simulink model "fengji"  (R2022b)
settings: Solver=VariableStepAuto  StartTime=0.0  StopTime=1.2  RelTol=1e-3
InitFcn:
  | Udc=311;
  | R=0.958;
  | Ld=5.25e-3;
  | Lq=12e-3;
  | flux=0.1827;
  | J=0.003;
  | B=0.008;
  | Pn=4;
  | Kpd=1100*0.958;
  | Kid=1100*R;
  | Kpq=1100*Lq;
  | Kiq=1100*R;
  | uppermin=-311*0.9*sqrt(1/3);
  | uppermax=311*0.9*sqrt(1/3);
  | uppermin2=-311*0.9*sqrt(1/3);
  | uppermax2=311*0.9*sqrt(1/3);
  | Kpw=0.14;
  | Kiw=0.14*50;
  | Ba=0.013;
undefined symbols (not defined in the file): DiscIntNeverNeededParam
libraries: simulink x11, slpidlib x6, spsabctodq0Lib x3, spsUniversalBridgeLib x3, spsPermanentMagnetSynchronousMachineLib x2, spsSVPWMGenerator2LevelLib x2, spsdq0toAlphaBetaZeroLib x2, spsPower3phInstantaneousLib x1, spsPower3phPhasorLib x1, spsSeriesRLCBranchLib x1, spsDCVoltageSourceLib x1, spsThreePhaseSeriesRLCBranchLib x1
(part 1 of 2)
settings Model: SimulationMode=accelerator  Creator=V V  LastModifiedBy=58239
settings SolverCC: AlgebraicLoopSolver=TrustRegion
settings OptimizationCC: LifeSpan=inf
settings DebuggingCC: UnconnectedInputMsg=warning  UnconnectedOutputMsg=warning  UnconnectedLineMsg=warning  SFExecutionAtInitializationDiag=none  SFMachineParentedDataDiag=warning  ArithmeticOperatorsInVariantConditions=warning
settings ModelReferenceCC: EnableRefExpFcnMdlSchedulingChecks=on
settings SFSimCC: CustomCodeUndefinedFunction=UseInterfaceOnly
settings CodeAppCC: StateflowObjectComments=on

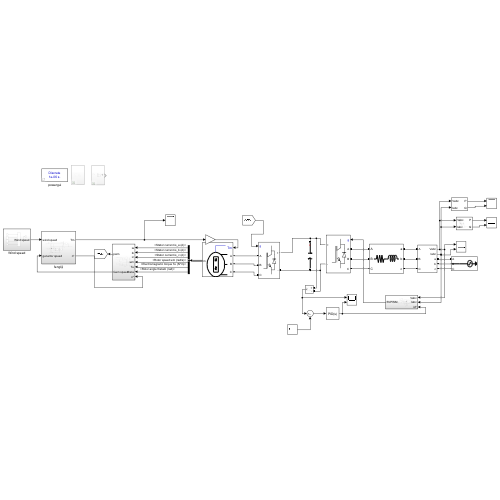
[thumbnail: Simulink's stored preview of the top-level diagram]
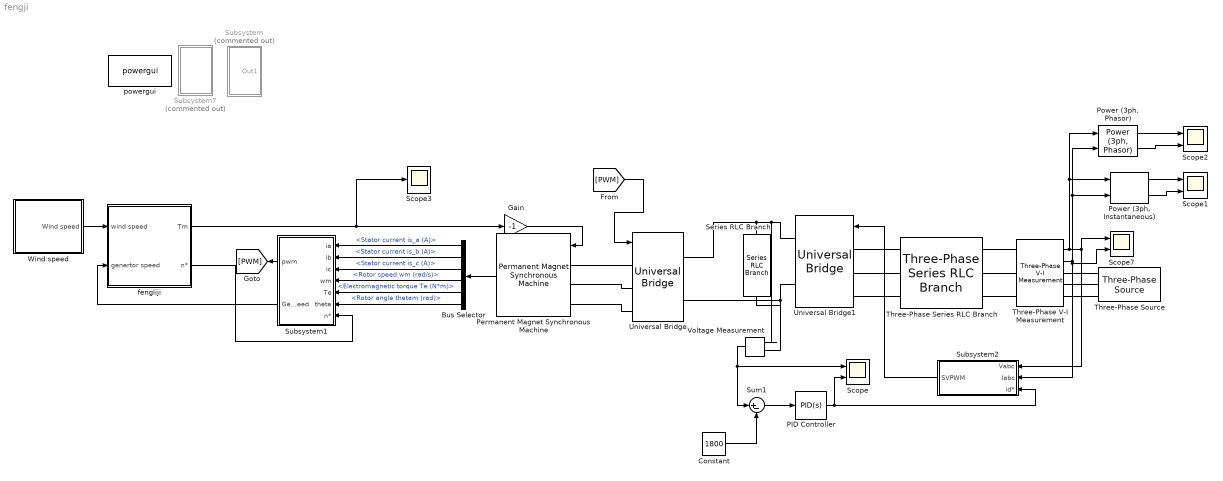
== system fengji ==
  Bus Selector : BusSelector  OutputSignals=Stator current is_a (A),Stator current is_b (A),Stator current is_c (A),Rotor speed wm (rad/s),Electromagnetic torque Te (N*m),Rotor angle thetam (rad)
  Constant : Constant  Value=1800
  Gain : Gain  Gain=-1
  PID Controller : slpidlib/PID Controller  Controller=PID  Form=Parallel  TimeDomain=Continuous-time  UseExternalTs=off  SampleTime=-1  IntegratorMethod=Forward Euler  FilterMethod=Forward Euler  ControllerParametersSource=internal  P=1  I=7  UseKiTs=off  D=0  N=100  UseFilter=on  TunerSelectOption=Transfer Function Based (PID Tuner App)  InitialConditionSource=internal  InitialConditionForIntegrator=0  InitialConditionForFilter=0  DifferentiatorICPrevScaledInput=0  ExternalReset=none  TrackingMode=off  Kt=1  LimitOutput=off  SatLimitsSource=internal  UpperSaturationLimit=inf  LowerSaturationLimit=-inf  LinearizeAsGain=on  AntiWindupMode=none  Kb=1  LimitIntegrator=off  UpperIntegratorSaturationLimit=inf  LowerIntegratorSaturationLimit=-inf  POutMin=[]  POutMax=[]  IOutMin=[]  IOutMax=[]  DOutMin=[]  DOutMax=[]  NOutMin=[]  NOutMax=[]  SumOutMin=[]  SumOutMax=[]  SaturationOutMin=[]  SaturationOutMax=[]  PParamMin=[]  PParamMax=[]  IParamMin=[]  IParamMax=[]  DParamMin=[]  DParamMax=[]  NParamMin=[]  NParamMax=[]  KbParamMin=[]  KbParamMax=[]  KtParamMin=[]  KtParamMax=[]  KbOutMin=[]  KbOutMax=[]  KtOutMin=[]  KtOutMax=[]  IntegratorOutMin=[]  IntegratorOutMax=[]  FilterOutMin=[]  FilterOutMax=[]  SumI1OutMin=[]  SumI1OutMax=[]  SumI2OutMin=[]  SumI2OutMax=[]  SumI3OutMin=[]  SumI3OutMax=[]  SumI4OutMin=[]  SumI4OutMax=[]  SumDOutMin=[]  SumDOutMax=[]  DifferentiatorOutMin=[]  DifferentiatorOutMax=[]  FilterDiffOutCoefMin=[]  FilterDiffOutCoefMax=[]  ReciprocalOutMin=[]  ReciprocalOutMax=[]  SumDenOutMin=[]  SumDenOutMax=[]  SumNumOutMin=[]  SumNumOutMax=[]  DivideOutMin=[]  DivideOutMax=[]  UdiffTsProdOutMin=[]  UdiffTsProdOutMax=[]  NTsProdOutMin=[]  NTsProdOutMax=[]  UintegralTsProdOutMin=[]  UintegralTsProdOutMax=[]  UngainTsProdOutMin=[]  UngainTsProdOutMax=[]  ClampingZeroOutDataTypeStr=Inherit: Inherit via back propagation  ClampingZeroOutMin=[]  ClampingZeroOutMax=[]  FilterDenConstantOutDataTypeStr=Inherit: Inherit via back propagation  FilterDenConstantOutMin=[]  FilterDenConstantOutMax=[]  PCopyOutDataTypeStr=Inherit: Inherit via back propagation  PCopyOutMin=[]  PCopyOutMax=[]  NCopyOutDataTypeStr=Inherit: Inherit via back propagation  NCopyOutMin=[]  NCopyOutMax=[]  IntegratorContinuousStateAttributes=''  IntegratorStateMustResolveToSignalObject=off  IntegratorRTWStateStorageClass=Auto  FilterContinuousStateAttributes=''  FilterStateMustResolveToSignalObject=off  FilterRTWStateStorageClass=Auto  ParallelPVariant=InternalParameters  IdealPVariant=Disabled  IVariant=InternalParameters  DVariant=InternalParameters  IntegratorVariant=Continuous  SatVariant=Disabled  AWVariant=Passthrough  PCopyVariant=Disabled  TRVariant=Disabled  FdbkBlocksVariant=Forward  IdealPFdbkVariant=Disabled  SatFdbkVariant=Disabled  DerivativeFilterVariant=ContFilter  NVariant=InternalParameters  NCopyVariant=Disabled  FilterICVariant=InternalICsFilter  IntegratorICVariant=InternalICs  ExternalResetVariant=Disabled  TRSumVariant=Passthrough  SumFdbkVariant=Disabled  SumVariant=Sum_PID  TsampFilterVariant=InternalTs  TsampNgainVariant=Passthrough  TsampIntegralVariant=Passthrough  ExternalSaturationOutDataTypeStr=Inherit: Same as second input
  Permanent Magnet Synchronous Machine : spsPermanentMagnetSynchronousMachineLib/Permanent Magnet Synchronous Machine  NbPhases=3  FluxDistribution=Sinusoidal  RotorType=Round  MechanicalLoad=Torque Tm  PresetModel=No  ShowDetailedParameters=on  MeasurementBus=off  Resistance=0.025  Inductance=8.5e-3  dqInductances=[8.5e-3,8.5e-3]  La=0.0036  MachineConstant=Flux linkage established by magnets (V.s)  Flux=3.88889  VoltageCst=8464.3995  TorqueCst=70  Flat=120  Mechanical=[60 0.078 12]  PolePairs=4  InitialConditions=[0,0, 0,0]  InitialConditions5ph=[0 0 0 0 0 0]  RefAngle=90 degrees behind phase A axis (modified Park)  IterativeDiscreteModel=Trapezoidal non iterative  TsBlock=-1  TsPowergui=0
  "Power (3ph, Instantaneous)" : spsPower3phInstantaneousLib/Power (3ph, Instantaneous)
  "Power (3ph, Phasor)" : spsPower3phPhasorLib/Power (3ph, Phasor)
      settings: LibrarySourceBlock=|
      | sps_lib/Sensors and Measurements/Power
      | (3ph, Phasor)
  Scope{,1..2,7} (4 alike) : Scope  NumInputPorts=2
  Scope3 : Scope
  Series RLC Branch : spsSeriesRLCBranchLib/Series RLC Branch  LConnTagsString=__new0  RConnTagsString=__new0  BranchType=C  Resistance=0.05  Inductance=1e-3  SetiL0=off  InitialCurrent=0  Capacitance=1e-2  Setx0=on  InitialVoltage=1800  Measurements=None
  Subsystem : Subsystem  Commented=on
  Subsystem1 : Subsystem
  Subsystem2 : Subsystem
  Subsystem7 : Subsystem  Commented=on
  Sum1 : Sum  Inputs=|+-
  Three-Phase Series RLC Branch : spsThreePhaseSeriesRLCBranchLib/Three-Phase Series RLC Branch  LConnTagsString=A|B|C  RConnTagsString=A|B|C  BranchType=RL  Resistance=0.05  Inductance=7e-3  Capacitance=1e-6  Measurements=None
  Three-Phase V-I Measurement : spsThreePhaseVIMeasurementLib/Three-Phase V-I Measurement  VoltageMeasurement=phase-to-ground  SetLabelV=off  LabelV=Vabc  Vpu=off  VpuLL=off  CurrentMeasurement=yes  SetLabelI=off  LabelI=Iabc  Ipu=off  Pbase=100e6  Vbase=500e3  OutputType=Complex  PhasorSimulation=off  PSBequivalent=0
  Three-Phase Source : spsThreePhaseSourceLib/Three-Phase Source  InternalConnection=Yg  VoltagePhases=off  Voltage=690  PhaseAngle=0  Voltage_phases=[25e3 25e3 25e3]/sqrt(3)  PhaseAngles_phases=[0 -120 +120]  Frequency=50  NonIdealSource=off  SpecifyImpedance=off  Resistance=0.8929  Inductance=16.58e-3  ShortCircuitLevel=100e6  BaseVoltage=25e3  XRratio=7  BusType=swing  Pref=10e3  Qref=0  Prefabc=[10e3, 10e3, 10e3]  Qrefabc=[0, 0, 0]  Qmin=-inf  Qmax=inf
  Universal Bridge : spsUniversalBridgeLib/Universal Bridge  Arms=3  SnubberResistance=1e5  SnubberCapacitance=inf  Device=IGBT / Diodes  Ron=1e-3  Lon=0  ForwardVoltages="[  0  0  ]"  ForwardVoltage=0  GTOparameters=[ 10e-6 , 20e-6 ]  IGBTparameters=[ 1e-6 , 2e-6 ]  Measurements=None  Measurements_2=None  converterType=Rectifier
  Universal Bridge1 : spsUniversalBridgeLib/Universal Bridge  Arms=3  SnubberResistance=1e5  SnubberCapacitance=inf  Device=IGBT / Diodes  Ron=1e-3  Lon=0  ForwardVoltages="[  0  0  ]"  ForwardVoltage=0  GTOparameters=[ 10e-6 , 20e-6 ]  IGBTparameters=[ 1e-6 , 2e-6 ]  Measurements=None  Measurements_2=None  converterType=Rectifier
  Voltage Measurement : spsVoltageMeasurementLib/Voltage Measurement  PhasorSimulation=off  OutputType=Complex  PSBequivalent=0
  Wind speed : Subsystem
  fengliji : Subsystem
  powergui : spspowerguiLib/powergui  Priority=1  SimulationMode=Discrete  SampleTime=1e-6  frequency=60  Iterations=50  frequencyindice=50  Pbase=100e6  ErrMax=1e-4  UnitsV=kV  UnitsW=MW  buscounter=0  FunctionMessages=off  echomessages=off  EnableUseOfTLC=off  CurrentSourceSwitches=off  DisableSnubberDevices=off  DisableRonSwitches=off  DisableVfSwitches=off  DisplayEquations=off  AutomaticDiscreteSolvers=off  SolverType=Tustin/Backward Euler (TBE)  Interpol=off  ExternalGateDelay=off  methode=off  Ts=100  x0status=blocks  SPID=on  SwTol=0  HookPort=off  NonlinearTolerance=1e-4  nMaxIteration=100  ContinueOnMaxIteration=off  RestoreLinks=warning  ResistiveCurrentMeasurement=off  Frange=[0:2:500]  Ylog=off  Xlog=on  ShowGrid=off  save=off  variable=ZData  structure=0  ZoomFFT=off  StartTime=0.0  cycles=1  DisplayStyle=1  fundamental=60  FreqAxis=off  MaxFrequency=1000  frequencyindicesteady=1  RmsSteady=1  display=off
  wires:
  Gain/1 -> Permanent Magnet Synchronous Machine/1
  Constant/1 -> Sum1/2
  Voltage Measurement/1 -> Sum1/1, Scope/1
  Sum1/1 -> PID Controller/1
  PID Controller/1 -> Subsystem2/3(id*), Scope/2
  [PWM] -> Universal Bridge/1
  fengliji/1(Tm) -> Scope3/1, Gain/1
  Permanent Magnet Synchronous Machine/1 -> Bus Selector/1
  Bus Selector/1 -> Subsystem1/1(ia)  "<Stator current is_a (A)>"
  Bus Selector/2 -> Subsystem1/2(ib)  "<Stator current is_b (A)>"
  Bus Selector/3 -> Subsystem1/3(ic)  "<Stator current is_c (A)>"
  fengliji/2(n*) -> Subsystem1/7(n*)
  Subsystem1/1(pwm) -> [PWM]
  Subsystem1/2(Gem speed) -> fengliji/2(genertor speed)
  Subsystem2/1(SVPWM) -> Universal Bridge1/1
  Three-Phase V-I Measurement/1 -> "Power (3ph, Instantaneous)"/1, "Power (3ph, Phasor)"/1, Scope7/1, Subsystem2/1(Vabc)
  Three-Phase V-I Measurement/2 -> "Power (3ph, Instantaneous)"/2, "Power (3ph, Phasor)"/2, Scope7/2, Subsystem2/2(Iabc)
  "Power (3ph, Phasor)"/2 -> Scope2/2
  "Power (3ph, Phasor)"/1 -> Scope2/1
  Bus Selector/4 -> Subsystem1/4(wm)  "<Rotor speed wm (rad/s)>"
  Bus Selector/5 -> Subsystem1/5(Te)  "<Electromagnetic torque Te (N*m)>"
  Bus Selector/6 -> Subsystem1/6(theta)  "<Rotor angle thetam (rad)>"
  "Power (3ph, Instantaneous)"/1 -> Scope1/1
  "Power (3ph, Instantaneous)"/2 -> Scope1/2
  Wind speed/1(Wind speed) -> fengliji/1(wind speed)
  connections:
  Universal Bridge1/RConn1 -- Voltage Measurement/LConn1 -- Universal Bridge/RConn1 -- Series RLC Branch/LConn1
  Series RLC Branch/RConn1 -- Universal Bridge/RConn2 -- Voltage Measurement/LConn2 -- Universal Bridge1/RConn2
  Three-Phase Series RLC Branch/LConn1 -- Universal Bridge1/LConn1
  Three-Phase Series RLC Branch/LConn2 -- Universal Bridge1/LConn2
  Three-Phase Series RLC Branch/LConn3 -- Universal Bridge1/LConn3
  Three-Phase V-I Measurement/LConn3 -- Three-Phase Series RLC Branch/RConn3
  Three-Phase V-I Measurement/LConn2 -- Three-Phase Series RLC Branch/RConn2
  Three-Phase V-I Measurement/LConn1 -- Three-Phase Series RLC Branch/RConn1
  Three-Phase Source/RConn1 -- Three-Phase V-I Measurement/RConn1
  Three-Phase Source/RConn2 -- Three-Phase V-I Measurement/RConn2
  Three-Phase Source/RConn3 -- Three-Phase V-I Measurement/RConn3
  Universal Bridge/LConn3 -- Permanent Magnet Synchronous Machine/LConn3
  Permanent Magnet Synchronous Machine/LConn2 -- Universal Bridge/LConn2
  Universal Bridge/LConn1 -- Permanent Magnet Synchronous Machine/LConn1

== system fengji/Subsystem ==
  Ramp : simulink/Sources/Ramp  slope=3  start=0  InitialOutput=0
  Step : Step  Commented=on  Time=1.5  After=-4  SampleTime=0
  Sum : Sum  Inputs=|++
  wind sp : Constant  Value=12
  Out1 : Outport
  wires:
  wind sp/1 -> Sum/1
  Ramp/1 -> Sum/2
  Sum/1 -> Out1/1

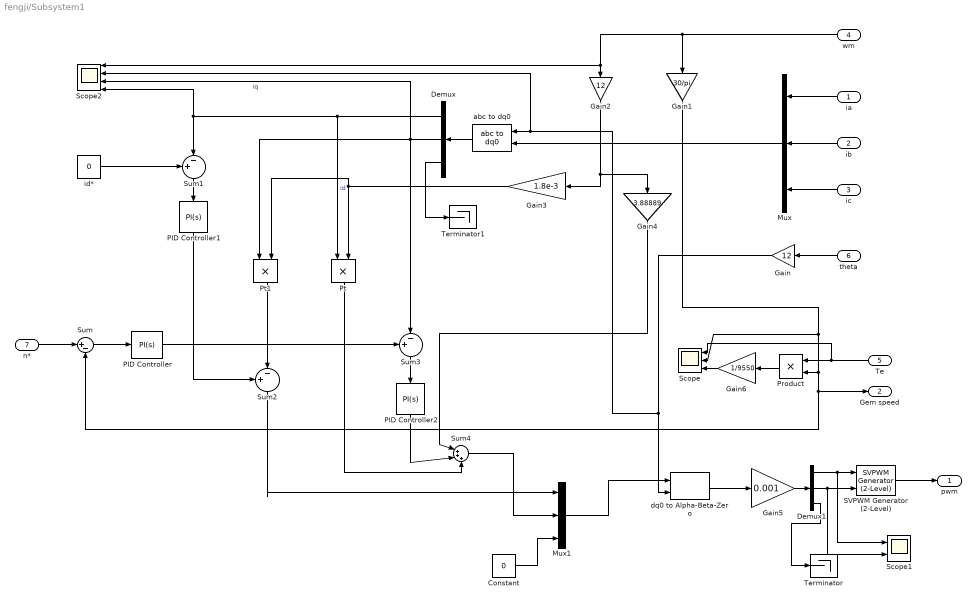
== system fengji/Subsystem1 ==
  ia : Inport
  ib : Inport  Port=2
  ic : Inport  Port=3
  wm : Inport  Port=4
  Te : Inport  Port=5
  theta : Inport  Port=6
  n* : Inport  Port=7
  Constant : Constant  Value=0
  Demux : Demux  Outputs=3
  Demux1 : Demux  Outputs=3
  Gain : Gain  Gain=12
  Gain1 : Gain  Gain=30/pi
  Gain2 : Gain  Gain=12
  Gain3 : Gain  Gain=1.8e-3
  Gain4 : Gain  Gain=3.88889
  Gain5 : Gain  Gain=0.001
  Gain6 : Gain  Gain=1/9550
  Mux : Mux  Inputs=3
  Mux1 : Mux  Inputs=3
  PID Controller : slpidlib/PID Controller  Controller=PI  Form=Parallel  TimeDomain=Continuous-time  UseExternalTs=off  SampleTime=-1  IntegratorMethod=Forward Euler  FilterMethod=Forward Euler  ControllerParametersSource=internal  P=10  I=220  UseKiTs=off  D=0  N=100  UseFilter=on  TunerSelectOption=Transfer Function Based (PID Tuner App)  InitialConditionSource=internal  InitialConditionForIntegrator=0  InitialConditionForFilter=0  DifferentiatorICPrevScaledInput=0  ExternalReset=none  TrackingMode=off  Kt=1  LimitOutput=off  SatLimitsSource=internal  UpperSaturationLimit=inf  LowerSaturationLimit=-inf  LinearizeAsGain=on  AntiWindupMode=none  Kb=1  LimitIntegrator=off  UpperIntegratorSaturationLimit=inf  LowerIntegratorSaturationLimit=-inf  POutMin=[]  POutMax=[]  IOutMin=[]  IOutMax=[]  DOutMin=[]  DOutMax=[]  NOutMin=[]  NOutMax=[]  SumOutMin=[]  SumOutMax=[]  SaturationOutMin=[]  SaturationOutMax=[]  PParamMin=[]  PParamMax=[]  IParamMin=[]  IParamMax=[]  DParamMin=[]  DParamMax=[]  NParamMin=[]  NParamMax=[]  KbParamMin=[]  KbParamMax=[]  KtParamMin=[]  KtParamMax=[]  KbOutMin=[]  KbOutMax=[]  KtOutMin=[]  KtOutMax=[]  IntegratorOutMin=[]  IntegratorOutMax=[]  FilterOutMin=[]  FilterOutMax=[]  SumI1OutMin=[]  SumI1OutMax=[]  SumI2OutMin=[]  SumI2OutMax=[]  SumI3OutMin=[]  SumI3OutMax=[]  SumI4OutMin=[]  SumI4OutMax=[]  SumDOutMin=[]  SumDOutMax=[]  DifferentiatorOutMin=[]  DifferentiatorOutMax=[]  FilterDiffOutCoefMin=[]  FilterDiffOutCoefMax=[]  ReciprocalOutMin=[]  ReciprocalOutMax=[]  SumDenOutMin=[]  SumDenOutMax=[]  SumNumOutMin=[]  SumNumOutMax=[]  DivideOutMin=[]  DivideOutMax=[]  UdiffTsProdOutMin=[]  UdiffTsProdOutMax=[]  NTsProdOutMin=[]  NTsProdOutMax=[]  UintegralTsProdOutMin=[]  UintegralTsProdOutMax=[]  UngainTsProdOutMin=[]  UngainTsProdOutMax=[]  ClampingZeroOutDataTypeStr=Inherit: Inherit via back propagation  ClampingZeroOutMin=[]  ClampingZeroOutMax=[]  FilterDenConstantOutDataTypeStr=Inherit: Inherit via back propagation  FilterDenConstantOutMin=[]  FilterDenConstantOutMax=[]  PCopyOutDataTypeStr=Inherit: Inherit via back propagation  PCopyOutMin=[]  PCopyOutMax=[]  NCopyOutDataTypeStr=Inherit: Inherit via back propagation  NCopyOutMin=[]  NCopyOutMax=[]  IntegratorContinuousStateAttributes=''  IntegratorStateMustResolveToSignalObject=off  IntegratorRTWStateStorageClass=Auto  FilterContinuousStateAttributes=''  FilterStateMustResolveToSignalObject=off  FilterRTWStateStorageClass=Auto  ParallelPVariant=InternalParameters  IdealPVariant=Disabled  IVariant=InternalParameters  DVariant=Disabled  IntegratorVariant=Continuous  SatVariant=Disabled  AWVariant=Passthrough  PCopyVariant=Disabled  TRVariant=Disabled  FdbkBlocksVariant=Forward  IdealPFdbkVariant=Disabled  SatFdbkVariant=Disabled  DerivativeFilterVariant=Disabled  NVariant=Disabled  NCopyVariant=Disabled_SignalSpec  FilterICVariant=Disabled  IntegratorICVariant=InternalICs  ExternalResetVariant=Disabled  TRSumVariant=Passthrough  SumFdbkVariant=Disabled  SumVariant=Sum_PI  TsampFilterVariant=InternalTs  TsampNgainVariant=Passthrough  TsampIntegralVariant=Passthrough  ExternalSaturationOutDataTypeStr=Inherit: Same as second input
  PID Controller1 : slpidlib/PID Controller  Controller=PI  Form=Parallel  TimeDomain=Continuous-time  UseExternalTs=off  SampleTime=-1  IntegratorMethod=Forward Euler  FilterMethod=Forward Euler  ControllerParametersSource=internal  P=1  I=12  UseKiTs=off  D=0  N=100  UseFilter=on  TunerSelectOption=Transfer Function Based (PID Tuner App)  InitialConditionSource=internal  InitialConditionForIntegrator=0  InitialConditionForFilter=0  DifferentiatorICPrevScaledInput=0  ExternalReset=none  TrackingMode=off  Kt=1  LimitOutput=off  SatLimitsSource=internal  UpperSaturationLimit=inf  LowerSaturationLimit=-inf  LinearizeAsGain=on  AntiWindupMode=none  Kb=1  LimitIntegrator=off  UpperIntegratorSaturationLimit=inf  LowerIntegratorSaturationLimit=-inf  POutMin=[]  POutMax=[]  IOutMin=[]  IOutMax=[]  DOutMin=[]  DOutMax=[]  NOutMin=[]  NOutMax=[]  SumOutMin=[]  SumOutMax=[]  SaturationOutMin=[]  SaturationOutMax=[]  PParamMin=[]  PParamMax=[]  IParamMin=[]  IParamMax=[]  DParamMin=[]  DParamMax=[]  NParamMin=[]  NParamMax=[]  KbParamMin=[]  KbParamMax=[]  KtParamMin=[]  KtParamMax=[]  KbOutMin=[]  KbOutMax=[]  KtOutMin=[]  KtOutMax=[]  IntegratorOutMin=[]  IntegratorOutMax=[]  FilterOutMin=[]  FilterOutMax=[]  SumI1OutMin=[]  SumI1OutMax=[]  SumI2OutMin=[]  SumI2OutMax=[]  SumI3OutMin=[]  SumI3OutMax=[]  SumI4OutMin=[]  SumI4OutMax=[]  SumDOutMin=[]  SumDOutMax=[]  DifferentiatorOutMin=[]  DifferentiatorOutMax=[]  FilterDiffOutCoefMin=[]  FilterDiffOutCoefMax=[]  ReciprocalOutMin=[]  ReciprocalOutMax=[]  SumDenOutMin=[]  SumDenOutMax=[]  SumNumOutMin=[]  SumNumOutMax=[]  DivideOutMin=[]  DivideOutMax=[]  UdiffTsProdOutMin=[]  UdiffTsProdOutMax=[]  NTsProdOutMin=[]  NTsProdOutMax=[]  UintegralTsProdOutMin=[]  UintegralTsProdOutMax=[]  UngainTsProdOutMin=[]  UngainTsProdOutMax=[]  ClampingZeroOutDataTypeStr=Inherit: Inherit via back propagation  ClampingZeroOutMin=[]  ClampingZeroOutMax=[]  FilterDenConstantOutDataTypeStr=Inherit: Inherit via back propagation  FilterDenConstantOutMin=[]  FilterDenConstantOutMax=[]  PCopyOutDataTypeStr=Inherit: Inherit via back propagation  PCopyOutMin=[]  PCopyOutMax=[]  NCopyOutDataTypeStr=Inherit: Inherit via back propagation  NCopyOutMin=[]  NCopyOutMax=[]  IntegratorContinuousStateAttributes=''  IntegratorStateMustResolveToSignalObject=off  IntegratorRTWStateStorageClass=Auto  FilterContinuousStateAttributes=''  FilterStateMustResolveToSignalObject=off  FilterRTWStateStorageClass=Auto  ParallelPVariant=InternalParameters  IdealPVariant=Disabled  IVariant=InternalParameters  DVariant=Disabled  IntegratorVariant=Continuous  SatVariant=Disabled  AWVariant=Passthrough  PCopyVariant=Disabled  TRVariant=Disabled  FdbkBlocksVariant=Forward  IdealPFdbkVariant=Disabled  SatFdbkVariant=Disabled  DerivativeFilterVariant=Disabled  NVariant=Disabled  NCopyVariant=Disabled_SignalSpec  FilterICVariant=Disabled  IntegratorICVariant=InternalICs  ExternalResetVariant=Disabled  TRSumVariant=Passthrough  SumFdbkVariant=Disabled  SumVariant=Sum_PI  TsampFilterVariant=InternalTs  TsampNgainVariant=Passthrough  TsampIntegralVariant=Passthrough  ExternalSaturationOutDataTypeStr=Inherit: Same as second input
  PID Controller2 : slpidlib/PID Controller  Controller=PI  Form=Parallel  TimeDomain=Continuous-time  UseExternalTs=off  SampleTime=-1  IntegratorMethod=Forward Euler  FilterMethod=Forward Euler  ControllerParametersSource=internal  P=1  I=12  UseKiTs=off  D=0  N=100  UseFilter=on  TunerSelectOption=Transfer Function Based (PID Tuner App)  InitialConditionSource=internal  InitialConditionForIntegrator=0  InitialConditionForFilter=0  DifferentiatorICPrevScaledInput=0  ExternalReset=none  TrackingMode=off  Kt=1  LimitOutput=off  SatLimitsSource=internal  UpperSaturationLimit=inf  LowerSaturationLimit=-inf  LinearizeAsGain=on  AntiWindupMode=none  Kb=1  LimitIntegrator=off  UpperIntegratorSaturationLimit=inf  LowerIntegratorSaturationLimit=-inf  POutMin=[]  POutMax=[]  IOutMin=[]  IOutMax=[]  DOutMin=[]  DOutMax=[]  NOutMin=[]  NOutMax=[]  SumOutMin=[]  SumOutMax=[]  SaturationOutMin=[]  SaturationOutMax=[]  PParamMin=[]  PParamMax=[]  IParamMin=[]  IParamMax=[]  DParamMin=[]  DParamMax=[]  NParamMin=[]  NParamMax=[]  KbParamMin=[]  KbParamMax=[]  KtParamMin=[]  KtParamMax=[]  KbOutMin=[]  KbOutMax=[]  KtOutMin=[]  KtOutMax=[]  IntegratorOutMin=[]  IntegratorOutMax=[]  FilterOutMin=[]  FilterOutMax=[]  SumI1OutMin=[]  SumI1OutMax=[]  SumI2OutMin=[]  SumI2OutMax=[]  SumI3OutMin=[]  SumI3OutMax=[]  SumI4OutMin=[]  SumI4OutMax=[]  SumDOutMin=[]  SumDOutMax=[]  DifferentiatorOutMin=[]  DifferentiatorOutMax=[]  FilterDiffOutCoefMin=[]  FilterDiffOutCoefMax=[]  ReciprocalOutMin=[]  ReciprocalOutMax=[]  SumDenOutMin=[]  SumDenOutMax=[]  SumNumOutMin=[]  SumNumOutMax=[]  DivideOutMin=[]  DivideOutMax=[]  UdiffTsProdOutMin=[]  UdiffTsProdOutMax=[]  NTsProdOutMin=[]  NTsProdOutMax=[]  UintegralTsProdOutMin=[]  UintegralTsProdOutMax=[]  UngainTsProdOutMin=[]  UngainTsProdOutMax=[]  ClampingZeroOutDataTypeStr=Inherit: Inherit via back propagation  ClampingZeroOutMin=[]  ClampingZeroOutMax=[]  FilterDenConstantOutDataTypeStr=Inherit: Inherit via back propagation  FilterDenConstantOutMin=[]  FilterDenConstantOutMax=[]  PCopyOutDataTypeStr=Inherit: Inherit via back propagation  PCopyOutMin=[]  PCopyOutMax=[]  NCopyOutDataTypeStr=Inherit: Inherit via back propagation  NCopyOutMin=[]  NCopyOutMax=[]  IntegratorContinuousStateAttributes=''  IntegratorStateMustResolveToSignalObject=off  IntegratorRTWStateStorageClass=Auto  FilterContinuousStateAttributes=''  FilterStateMustResolveToSignalObject=off  FilterRTWStateStorageClass=Auto  ParallelPVariant=InternalParameters  IdealPVariant=Disabled  IVariant=InternalParameters  DVariant=Disabled  IntegratorVariant=Continuous  SatVariant=Disabled  AWVariant=Passthrough  PCopyVariant=Disabled  TRVariant=Disabled  FdbkBlocksVariant=Forward  IdealPFdbkVariant=Disabled  SatFdbkVariant=Disabled  DerivativeFilterVariant=Disabled  NVariant=Disabled  NCopyVariant=Disabled_SignalSpec  FilterICVariant=Disabled  IntegratorICVariant=InternalICs  ExternalResetVariant=Disabled  TRSumVariant=Passthrough  SumFdbkVariant=Disabled  SumVariant=Sum_PI  TsampFilterVariant=InternalTs  TsampNgainVariant=Passthrough  TsampIntegralVariant=Passthrough  ExternalSaturationOutDataTypeStr=Inherit: Same as second input
  Product : Product
  Pt : Product
  Pt1 : Product
  SVPWM Generator (2-Level) : spsSVPWMGenerator2LevelLib/SVPWM Generator (2-Level)  InputType=alpha-beta components  SwitchingPattern=Pattern #1  Fc=3000  ParUref=[0.8 -30 50]  Ts=0
  Scope : Scope  NumInputPorts=3
  Scope1 : Scope  NumInputPorts=2
  Scope2 : Scope  NumInputPorts=4
  Sum : Sum  Inputs=|+-
  Sum1 : Sum  Inputs=+-|
  Sum2 : Sum  Inputs=+-|
  Sum3 : Sum  Inputs=+-|
  Sum4 : Sum  Inputs=|+++
  Terminator : Terminator
  Terminator1 : Terminator
  abc to dq0 : spsabctodq0Lib/abc to dq0  Alignment=90 degrees behind phase A axis
  dq0 to Alpha-Beta-Zero : spsdq0toAlphaBetaZeroLib/dq0 to Alpha-Beta-Zero  Alignment=90 degrees behind phase A axis
  id* : Constant  Value=0
  pwm : Outport
  Gem speed : Outport  Port=2
  wires:
  Mux1/1 -> dq0 to Alpha-Beta-Zero/1
  PID Controller1/1 -> Sum2/1
  abc to dq0/1 -> Demux/1
  Gain5/1 -> Demux1/1
  Sum2/1 -> Mux1/1
  Pt/1 -> Sum4/3
  PID Controller2/1 -> Sum4/2
  Sum4/1 -> Mux1/2
  Constant/1 -> Mux1/3
  Demux/2 -> Scope2/3, Pt1/1, Sum3/2  "iq"
  Demux/1 -> Scope2/4, Sum1/2, Pt/1  "id"
  Sum3/1 -> PID Controller2/1
  Demux1/1 -> Scope1/1, SVPWM Generator (2-Level)/1
  Pt1/1 -> Sum2/2
  id*/1 -> Sum1/1
  Gain4/1 -> Sum4/1
  Sum1/1 -> PID Controller1/1
  Gain/1 -> Scope2/2, abc to dq0/2, dq0 to Alpha-Beta-Zero/2
  Gain2/1 -> Gain4/1, Gain3/1
  Gain3/1 -> Pt1/2, Pt/2
  Mux/1 -> abc to dq0/1
  dq0 to Alpha-Beta-Zero/1 -> Gain5/1
  n*/1 -> Sum/1
  wm/1 -> Scope2/1, Gain2/1, Gain1/1
  PID Controller/1 -> Sum3/1
  Demux1/2 -> Scope1/2, SVPWM Generator (2-Level)/2
  ib/1 -> Mux/2
  Demux1/3 -> Terminator/1
  ic/1 -> Mux/3
  theta/1 -> Gain/1
  Sum/1 -> PID Controller/1
  ia/1 -> Mux/1
  SVPWM Generator (2-Level)/1 -> pwm/1
  Gain6/1 -> Scope/3
  Product/1 -> Gain6/1
  Gain1/1 -> Scope/2, Sum/2, Gem speed/1, Product/2
  Te/1 -> Scope/1, Product/1
  Demux/3 -> Terminator1/1

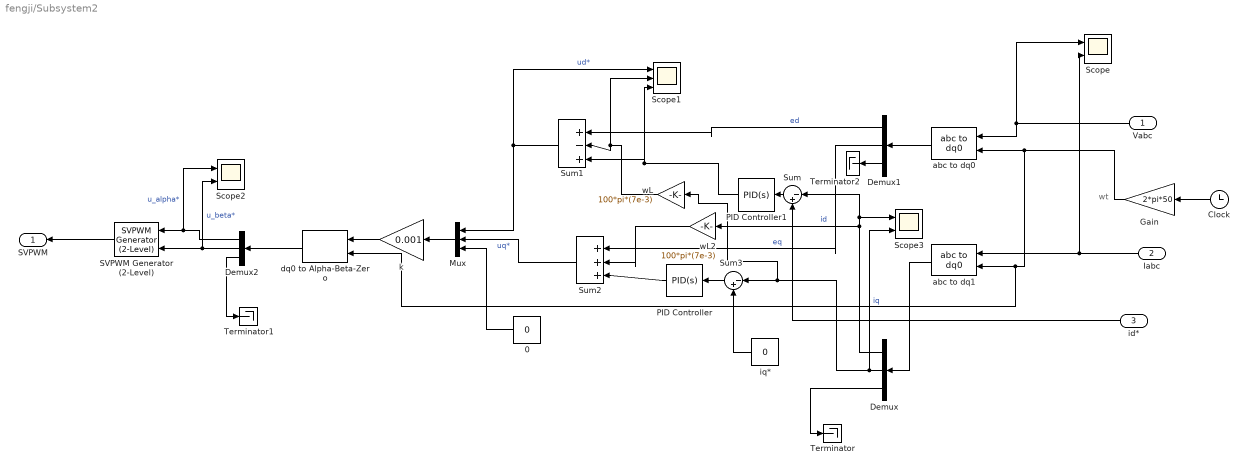
== system fengji/Subsystem2 ==
  note: wt
  Vabc : Inport
  Iabc : Inport  Port=2
  id* : Inport  Port=3
  0 : Constant  Value=0
  Clock : Clock
  Demux : Demux  Outputs=3
  Demux1 : Demux  Outputs=3
  Demux2 : Demux  Outputs=3
  Gain : Gain  Gain=2*pi*50
  Mux : Mux  Inputs=3
  PID Controller : slpidlib/PID Controller  Controller=PID  Form=Parallel  TimeDomain=Continuous-time  UseExternalTs=off  SampleTime=-1  IntegratorMethod=Forward Euler  FilterMethod=Forward Euler  ControllerParametersSource=internal  P=1  I=15  UseKiTs=off  D=0  N=100  UseFilter=on  TunerSelectOption=Transfer Function Based (PID Tuner App)  InitialConditionSource=internal  InitialConditionForIntegrator=0  InitialConditionForFilter=0  DifferentiatorICPrevScaledInput=0  ExternalReset=none  TrackingMode=off  Kt=1  LimitOutput=off  SatLimitsSource=internal  UpperSaturationLimit=inf  LowerSaturationLimit=-inf  LinearizeAsGain=on  AntiWindupMode=none  Kb=1  LimitIntegrator=off  UpperIntegratorSaturationLimit=inf  LowerIntegratorSaturationLimit=-inf  POutMin=[]  POutMax=[]  IOutMin=[]  IOutMax=[]  DOutMin=[]  DOutMax=[]  NOutMin=[]  NOutMax=[]  SumOutMin=[]  SumOutMax=[]  SaturationOutMin=[]  SaturationOutMax=[]  PParamMin=[]  PParamMax=[]  IParamMin=[]  IParamMax=[]  DParamMin=[]  DParamMax=[]  NParamMin=[]  NParamMax=[]  KbParamMin=[]  KbParamMax=[]  KtParamMin=[]  KtParamMax=[]  KbOutMin=[]  KbOutMax=[]  KtOutMin=[]  KtOutMax=[]  IntegratorOutMin=[]  IntegratorOutMax=[]  FilterOutMin=[]  FilterOutMax=[]  SumI1OutMin=[]  SumI1OutMax=[]  SumI2OutMin=[]  SumI2OutMax=[]  SumI3OutMin=[]  SumI3OutMax=[]  SumI4OutMin=[]  SumI4OutMax=[]  SumDOutMin=[]  SumDOutMax=[]  DifferentiatorOutMin=[]  DifferentiatorOutMax=[]  FilterDiffOutCoefMin=[]  FilterDiffOutCoefMax=[]  ReciprocalOutMin=[]  ReciprocalOutMax=[]  SumDenOutMin=[]  SumDenOutMax=[]  SumNumOutMin=[]  SumNumOutMax=[]  DivideOutMin=[]  DivideOutMax=[]  UdiffTsProdOutMin=[]  UdiffTsProdOutMax=[]  NTsProdOutMin=[]  NTsProdOutMax=[]  UintegralTsProdOutMin=[]  UintegralTsProdOutMax=[]  UngainTsProdOutMin=[]  UngainTsProdOutMax=[]  ClampingZeroOutDataTypeStr=Inherit: Inherit via back propagation  ClampingZeroOutMin=[]  ClampingZeroOutMax=[]  FilterDenConstantOutDataTypeStr=Inherit: Inherit via back propagation  FilterDenConstantOutMin=[]  FilterDenConstantOutMax=[]  PCopyOutDataTypeStr=Inherit: Inherit via back propagation  PCopyOutMin=[]  PCopyOutMax=[]  NCopyOutDataTypeStr=Inherit: Inherit via back propagation  NCopyOutMin=[]  NCopyOutMax=[]  IntegratorContinuousStateAttributes=''  IntegratorStateMustResolveToSignalObject=off  IntegratorRTWStateStorageClass=Auto  FilterContinuousStateAttributes=''  FilterStateMustResolveToSignalObject=off  FilterRTWStateStorageClass=Auto  ParallelPVariant=InternalParameters  IdealPVariant=Disabled  IVariant=InternalParameters  DVariant=InternalParameters  IntegratorVariant=Continuous  SatVariant=Disabled  AWVariant=Passthrough  PCopyVariant=Disabled  TRVariant=Disabled  FdbkBlocksVariant=Forward  IdealPFdbkVariant=Disabled  SatFdbkVariant=Disabled  DerivativeFilterVariant=ContFilter  NVariant=InternalParameters  NCopyVariant=Disabled  FilterICVariant=InternalICsFilter  IntegratorICVariant=InternalICs  ExternalResetVariant=Disabled  TRSumVariant=Passthrough  SumFdbkVariant=Disabled  SumVariant=Sum_PID  TsampFilterVariant=InternalTs  TsampNgainVariant=Passthrough  TsampIntegralVariant=Passthrough  ExternalSaturationOutDataTypeStr=Inherit: Same as second input
  PID Controller1 : slpidlib/PID Controller  Controller=PID  Form=Parallel  TimeDomain=Continuous-time  UseExternalTs=off  SampleTime=-1  IntegratorMethod=Forward Euler  FilterMethod=Forward Euler  ControllerParametersSource=internal  P=1  I=15  UseKiTs=off  D=0  N=100  UseFilter=on  TunerSelectOption=Transfer Function Based (PID Tuner App)  InitialConditionSource=internal  InitialConditionForIntegrator=0  InitialConditionForFilter=0  DifferentiatorICPrevScaledInput=0  ExternalReset=none  TrackingMode=off  Kt=1  LimitOutput=off  SatLimitsSource=internal  UpperSaturationLimit=inf  LowerSaturationLimit=-inf  LinearizeAsGain=on  AntiWindupMode=none  Kb=1  LimitIntegrator=off  UpperIntegratorSaturationLimit=inf  LowerIntegratorSaturationLimit=-inf  POutMin=[]  POutMax=[]  IOutMin=[]  IOutMax=[]  DOutMin=[]  DOutMax=[]  NOutMin=[]  NOutMax=[]  SumOutMin=[]  SumOutMax=[]  SaturationOutMin=[]  SaturationOutMax=[]  PParamMin=[]  PParamMax=[]  IParamMin=[]  IParamMax=[]  DParamMin=[]  DParamMax=[]  NParamMin=[]  NParamMax=[]  KbParamMin=[]  KbParamMax=[]  KtParamMin=[]  KtParamMax=[]  KbOutMin=[]  KbOutMax=[]  KtOutMin=[]  KtOutMax=[]  IntegratorOutMin=[]  IntegratorOutMax=[]  FilterOutMin=[]  FilterOutMax=[]  SumI1OutMin=[]  SumI1OutMax=[]  SumI2OutMin=[]  SumI2OutMax=[]  SumI3OutMin=[]  SumI3OutMax=[]  SumI4OutMin=[]  SumI4OutMax=[]  SumDOutMin=[]  SumDOutMax=[]  DifferentiatorOutMin=[]  DifferentiatorOutMax=[]  FilterDiffOutCoefMin=[]  FilterDiffOutCoefMax=[]  ReciprocalOutMin=[]  ReciprocalOutMax=[]  SumDenOutMin=[]  SumDenOutMax=[]  SumNumOutMin=[]  SumNumOutMax=[]  DivideOutMin=[]  DivideOutMax=[]  UdiffTsProdOutMin=[]  UdiffTsProdOutMax=[]  NTsProdOutMin=[]  NTsProdOutMax=[]  UintegralTsProdOutMin=[]  UintegralTsProdOutMax=[]  UngainTsProdOutMin=[]  UngainTsProdOutMax=[]  ClampingZeroOutDataTypeStr=Inherit: Inherit via back propagation  ClampingZeroOutMin=[]  ClampingZeroOutMax=[]  FilterDenConstantOutDataTypeStr=Inherit: Inherit via back propagation  FilterDenConstantOutMin=[]  FilterDenConstantOutMax=[]  PCopyOutDataTypeStr=Inherit: Inherit via back propagation  PCopyOutMin=[]  PCopyOutMax=[]  NCopyOutDataTypeStr=Inherit: Inherit via back propagation  NCopyOutMin=[]  NCopyOutMax=[]  IntegratorContinuousStateAttributes=''  IntegratorStateMustResolveToSignalObject=off  IntegratorRTWStateStorageClass=Auto  FilterContinuousStateAttributes=''  FilterStateMustResolveToSignalObject=off  FilterRTWStateStorageClass=Auto  ParallelPVariant=InternalParameters  IdealPVariant=Disabled  IVariant=InternalParameters  DVariant=InternalParameters  IntegratorVariant=Continuous  SatVariant=Disabled  AWVariant=Passthrough  PCopyVariant=Disabled  TRVariant=Disabled  FdbkBlocksVariant=Forward  IdealPFdbkVariant=Disabled  SatFdbkVariant=Disabled  DerivativeFilterVariant=ContFilter  NVariant=InternalParameters  NCopyVariant=Disabled  FilterICVariant=InternalICsFilter  IntegratorICVariant=InternalICs  ExternalResetVariant=Disabled  TRSumVariant=Passthrough  SumFdbkVariant=Disabled  SumVariant=Sum_PID  TsampFilterVariant=InternalTs  TsampNgainVariant=Passthrough  TsampIntegralVariant=Passthrough  ExternalSaturationOutDataTypeStr=Inherit: Same as second input
  SVPWM Generator (2-Level) : spsSVPWMGenerator2LevelLib/SVPWM Generator (2-Level)  InputType=alpha-beta components  SwitchingPattern=Pattern #1  Fc=3000  ParUref=[0.8 -30 50]  Ts=0
  Scope : Scope  NumInputPorts=2
  Scope1 : Scope  NumInputPorts=3
  Scope2 : Scope  NumInputPorts=2
  Scope3 : Scope  NumInputPorts=2
  Sum : Sum  Inputs=|-+
  Sum1 : Sum  Inputs=|+-+
  Sum2 : Sum  Inputs=|+++
  Sum3 : Sum  Inputs=|-+
  Terminator : Terminator
  Terminator1 : Terminator
  Terminator2 : Terminator
  abc to dq0 : spsabctodq0Lib/abc to dq0  Alignment=90 degrees behind phase A axis
  abc to dq1 : spsabctodq0Lib/abc to dq0  Alignment=90 degrees behind phase A axis
  dq0 to Alpha-Beta-Zero : spsdq0toAlphaBetaZeroLib/dq0 to Alpha-Beta-Zero  Alignment=90 degrees behind phase A axis
  iq* : Constant  Value=0
  k : Gain  Gain=0.001
  wL : Gain  Gain=100*pi*(7e-3)
  wL2 : Gain  Gain=100*pi*(7e-3)
  SVPWM : Outport
  wires:
  Clock/1 -> Gain/1
  Vabc/1 -> Scope/1, abc to dq0/1
  Gain/1 -> dq0 to Alpha-Beta-Zero/2, abc to dq1/2, abc to dq0/2
  Iabc/1 -> Scope/2, abc to dq1/1
  abc to dq1/1 -> Demux/1
  abc to dq0/1 -> Demux1/1
  Demux1/1 -> Sum1/1  "ed"
  Demux/1 -> Scope3/1, Sum/1, wL2/1  "id"
  id*/1 -> Sum/2
  iq*/1 -> Sum3/2
  Sum3/1 -> PID Controller/1
  PID Controller/1 -> Sum2/3
  wL2/1 -> Sum2/2
  Demux1/2 -> Sum2/1  "eq"
  Demux/2 -> Scope3/2, wL/1, Sum3/1  "iq"
  Demux/3 -> Terminator/1
  Sum/1 -> PID Controller1/1
  PID Controller1/1 -> Scope1/3, Sum1/3
  wL/1 -> Scope1/2, Sum1/2
  Sum1/1 -> Scope1/1, Mux/1  "ud*"
  Sum2/1 -> Mux/2  "uq*"
  0/1 -> Mux/3
  Mux/1 -> k/1
  dq0 to Alpha-Beta-Zero/1 -> Demux2/1
  Demux2/2 -> Scope2/2, SVPWM Generator (2-Level)/2  "u_beta*"
  Demux2/1 -> Scope2/1, SVPWM Generator (2-Level)/1  "u_alpha*"
  SVPWM Generator (2-Level)/1 -> SVPWM/1
  Demux2/3 -> Terminator1/1
  k/1 -> dq0 to Alpha-Beta-Zero/1
  Demux1/3 -> Terminator2/1

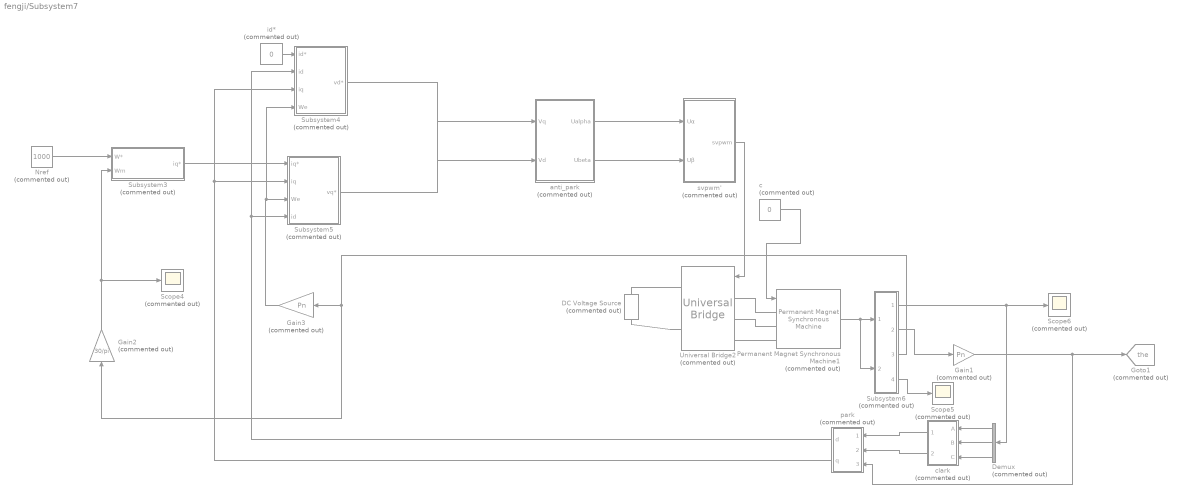
== system fengji/Subsystem7 ==
  DC Voltage Source : spsDCVoltageSourceLib/DC Voltage Source  Commented=on  Amplitude=Udc  Measurements=None
  Demux : Demux  Commented=on  Outputs=3
  Gain1 : Gain  Commented=on  Gain=Pn
  Gain2 : Gain  Commented=on  Gain=30/pi
  Gain3 : Gain  Commented=on  Gain=Pn
  Goto1 : Goto  Commented=on  GotoTag=the  TagVisibility=global
  Nref : Constant  Commented=on  Value=1000
  Permanent Magnet Synchronous Machine1 : spsPermanentMagnetSynchronousMachineLib/Permanent Magnet Synchronous Machine  Commented=on  NbPhases=3  FluxDistribution=Sinusoidal  RotorType=Salient-pole  MechanicalLoad=Torque Tm  PresetModel=No  ShowDetailedParameters=on  MeasurementBus=off  Resistance=R  Inductance=8.5e-3  dqInductances=[Ld,Lq]  La=0.000395  MachineConstant=Flux linkage established by magnets (V.s)  Flux=flux  VoltageCst=132.5525  TorqueCst=1.0962  Flat=120  Mechanical=[J B Pn 0]  PolePairs=4  InitialConditions=[0,0, 0,0]  InitialConditions5ph=[0 0 0 0 0 0]  RefAngle=Aligned with phase A axis (original Park)  IterativeDiscreteModel=Trapezoidal non iterative  TsBlock=-1  TsPowergui=0
  Scope4 : Scope  Commented=on
  Scope5 : Scope  Commented=on
  Scope6 : Scope  Commented=on
  Subsystem3 : Subsystem  Commented=on
  Subsystem4 : Subsystem  Commented=on
  Subsystem5 : Subsystem  Commented=on
  Subsystem6 : Subsystem  Commented=on
  Universal Bridge2 : spsUniversalBridgeLib/Universal Bridge  Commented=on  Arms=3  SnubberResistance=1e5  SnubberCapacitance=inf  Device=IGBT / Diodes  Ron=1e-3  Lon=0  ForwardVoltages="[  0  0  ]"  ForwardVoltage=0  GTOparameters=[ 10e-6 , 20e-6 ]  IGBTparameters=[ 1e-6 , 2e-6 ]  Measurements=None  Measurements_2=None  converterType=Rectifier
  anti_park : Subsystem  Commented=on
  c : Constant  Commented=on  Value=0
  clark : Subsystem  Commented=on
  id* : Constant  Commented=on  Value=0
  park : Subsystem  Commented=on
  svpwm' : Subsystem  Commented=on
  wires:
  Subsystem6/2(theta) -> Gain1/1
  Subsystem6/3(Wm) -> Gain2/1, Gain3/1
  clark/1(Alpha) -> park/1(Alpha1)
  Subsystem5/1(vq*) -> anti_park/1(Vq)
  Subsystem6/1(iabc) -> Scope6/1, Demux/1
  Gain2/1 -> Scope4/1, Subsystem3/2(Wm)
  svpwm'/1(svpwm) -> Universal Bridge2/1
  anti_park/1(Ualpha) -> svpwm'/1(Uα)
  Demux/2 -> clark/2(B)
  Subsystem6/4(Te) -> Scope5/1
  Subsystem3/1(iq*) -> Subsystem5/1(iq*)
  Demux/1 -> clark/1(A)
  park/1(d) -> Subsystem5/4(id), Subsystem4/2(id)
  park/2(q) -> Subsystem5/2(iq), Subsystem4/3(iq)
  Demux/3 -> clark/3(C)
  anti_park/2(Ubeta) -> svpwm'/2(Uβ)
  Subsystem4/1(vd*) -> anti_park/2(Vd)
  Gain3/1 -> Subsystem4/4(We), Subsystem5/3(We)
  id*/1 -> Subsystem4/1(id*)
  Nref/1 -> Subsystem3/1(W*)
  c/1 -> Permanent Magnet Synchronous Machine1/1
  clark/2(Beta) -> park/2(Beta1)
  Permanent Magnet Synchronous Machine1/1 -> Subsystem6/2(In2), Subsystem6/1(In1)
  Gain1/1 -> Goto1/1, park/3(theta)
  connections:
  Universal Bridge2/RConn2 -- DC Voltage Source/LConn1
  Permanent Magnet Synchronous Machine1/LConn1 -- Universal Bridge2/LConn1
  Permanent Magnet Synchronous Machine1/LConn2 -- Universal Bridge2/LConn2
  Universal Bridge2/RConn1 -- DC Voltage Source/RConn1
  Permanent Magnet Synchronous Machine1/LConn3 -- Universal Bridge2/LConn3

== system fengji/Wind speed ==
  Add : Sum  Inputs=++++
  Basic wind : Constant  Value=8
  Random Number : RandomNumber  Variance=0.3  SampleTime=0.02
  Scope : Scope
  jianbianfeng : Subsystem
  zhenfeng : Subsystem
  Wind speed : Outport
  wires:
  jianbianfeng/1(Vwr) -> Add/3
  Random Number/1 -> Add/4
  Basic wind/1 -> Add/1
  zhenfeng/1(Vwg) -> Add/2
  Add/1 -> Scope/1, Wind speed/1

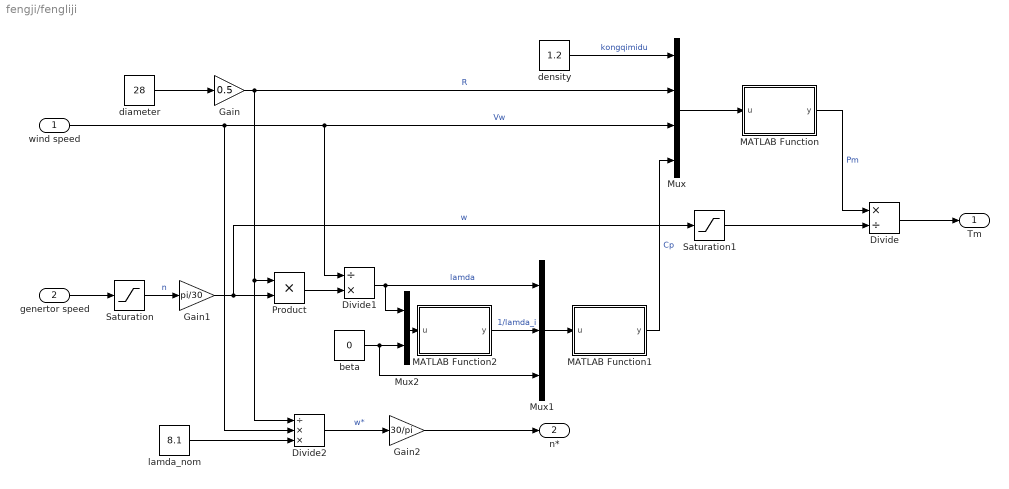
== system fengji/fengliji ==
  wind speed : Inport
  genertor speed : Inport  Port=2
  Divide : Product  Inputs=*/
  Divide1 : Product  Inputs=/*
  Divide2 : Product  Inputs=/**
  Gain : Gain  Gain=0.5
  Gain1 : Gain  Gain=pi/30
  Gain2 : Gain  Gain=30/pi
  MATLAB Function : MATLAB Function  TreatAsAtomicUnit=on
  MATLAB Function1 : MATLAB Function  TreatAsAtomicUnit=on
  MATLAB Function2 : MATLAB Function  TreatAsAtomicUnit=on
  Mux : Mux
  Mux1 : Mux  Inputs=3
  Mux2 : Mux  Inputs=2
  Product : Product
  Saturation : Saturate  UpperLimit=1e6  LowerLimit=1e-6
  Saturation1 : Saturate  UpperLimit=1e6  LowerLimit=1e-6
  beta : Constant  Value=0
  density : Constant  Value=1.2
  diameter : Constant  Value=28
  lamda_nom : Constant  Value=8.1
  Tm : Outport
  n* : Outport  Port=2
  wires:
  diameter/1 -> Gain/1
  density/1 -> Mux/1  "kongqimidu"
  Gain/1 -> Mux/2, Divide2/1, Product/1  "R"
  wind speed/1 -> Divide2/2, Mux/3, Divide1/1  "Vw"
  genertor speed/1 -> Saturation/1
  Saturation/1 -> Gain1/1  "n"
  Gain1/1 -> Saturation1/1, Product/2  "w"
  Saturation1/1 -> Divide/2
  Mux/1 -> MATLAB Function/1(u)
  MATLAB Function/1(y) -> Divide/1  "Pm"
  Divide/1 -> Tm/1
  MATLAB Function1/1(y) -> Mux/4  "Cp"
  Mux1/1 -> MATLAB Function1/1(u)
  Product/1 -> Divide1/2
  Divide1/1 -> Mux2/1, Mux1/1  "lamda"
  Mux2/1 -> MATLAB Function2/1(u)
  beta/1 -> Mux1/3, Mux2/2
  MATLAB Function2/1(y) -> Mux1/2  "1/lamda_i"
  Divide2/1 -> Gain2/1  "w*"
  Gain2/1 -> n*/1
  lamda_nom/1 -> Divide2/3

== system fengji/Subsystem7/Subsystem3 ==
  W* : Inport
  Wm : Inport  Port=2
  Discrete-Time Integrator : DiscreteIntegrator  SampleTime=-1  ICPrevOutput=DiscIntNeverNeededParam  ICPrevScaledInput=DiscIntNeverNeededParam
  Gain : Gain  Gain=Kpw
  Gain2 : Gain  Gain=Ba
  Gain4 : Gain  Gain=Kiw
  Saturation1 : Saturate  UpperLimit=30  LowerLimit=-30
  Sum : Sum  Inputs=|+-
  Sum1 : Sum  Inputs=|++
  Sum2 : Sum  Inputs=|+-
  Zero-Order Hold : ZeroOrderHold  SampleTime=-1
  iq* : Outport
  wires:
  Gain/1 -> Zero-Order Hold/1
  Sum/1 -> Gain4/1, Gain/1
  Zero-Order Hold/1 -> Sum1/1
  Discrete-Time Integrator/1 -> Sum1/2
  Sum1/1 -> Sum2/1
  Gain2/1 -> Sum2/2
  Sum2/1 -> Saturation1/1
  Saturation1/1 -> iq*/1
  Gain4/1 -> Discrete-Time Integrator/1
  Wm/1 -> Gain2/1, Sum/2
  W*/1 -> Sum/1

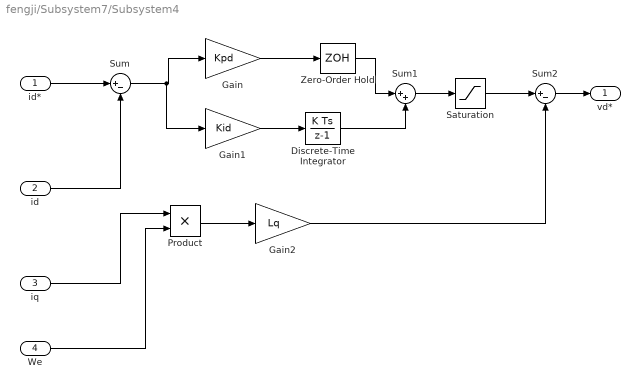
== system fengji/Subsystem7/Subsystem4 ==
  id* : Inport
  id : Inport  Port=2
  iq : Inport  Port=3
  We : Inport  Port=4
  Discrete-Time Integrator : DiscreteIntegrator  SampleTime=-1  ICPrevOutput=DiscIntNeverNeededParam  ICPrevScaledInput=DiscIntNeverNeededParam
  Gain : Gain  Gain=Kpd
  Gain1 : Gain  Gain=Kid
  Gain2 : Gain  Gain=Lq
  Product : Product
  Saturation : Saturate  UpperLimit=uppermax  LowerLimit=uppermin
  Sum : Sum  Inputs=|+-
  Sum1 : Sum  Inputs=|++
  Sum2 : Sum  Inputs=|+-
  Zero-Order Hold : ZeroOrderHold  SampleTime=-1
  vd* : Outport
  wires:
  Sum2/1 -> vd*/1
  Gain2/1 -> Sum2/2
  Saturation/1 -> Sum2/1
  Sum1/1 -> Saturation/1
  Discrete-Time Integrator/1 -> Sum1/2
  Zero-Order Hold/1 -> Sum1/1
  Sum/1 -> Gain/1, Gain1/1
  Gain1/1 -> Discrete-Time Integrator/1
  Gain/1 -> Zero-Order Hold/1
  id/1 -> Sum/2
  id*/1 -> Sum/1
  iq/1 -> Product/1
  Product/1 -> Gain2/1
  We/1 -> Product/2

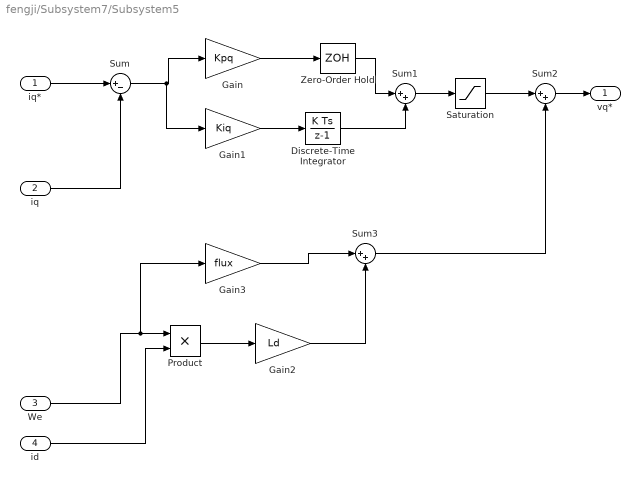
== system fengji/Subsystem7/Subsystem5 ==
  iq* : Inport
  iq : Inport  Port=2
  We : Inport  Port=3
  id : Inport  Port=4
  Discrete-Time Integrator : DiscreteIntegrator  SampleTime=-1  ICPrevOutput=DiscIntNeverNeededParam  ICPrevScaledInput=DiscIntNeverNeededParam
  Gain : Gain  Gain=Kpq
  Gain1 : Gain  Gain=Kiq
  Gain2 : Gain  Gain=Ld
  Gain3 : Gain  Gain=flux
  Product : Product
  Saturation : Saturate  UpperLimit=uppermax2  LowerLimit=uppermin2
  Sum : Sum  Inputs=|+-
  Sum1 : Sum  Inputs=|++
  Sum2 : Sum  Inputs=|++
  Sum3 : Sum  Inputs=|++
  Zero-Order Hold : ZeroOrderHold  SampleTime=-1
  vq* : Outport
  wires:
  id/1 -> Product/2
  Product/1 -> Gain2/1
  We/1 -> Gain3/1, Product/1
  iq*/1 -> Sum/1
  iq/1 -> Sum/2
  Gain/1 -> Zero-Order Hold/1
  Gain1/1 -> Discrete-Time Integrator/1
  Sum/1 -> Gain1/1, Gain/1
  Zero-Order Hold/1 -> Sum1/1
  Discrete-Time Integrator/1 -> Sum1/2
  Sum1/1 -> Saturation/1
  Saturation/1 -> Sum2/1
  Sum2/1 -> vq*/1
  Gain3/1 -> Sum3/1
  Gain2/1 -> Sum3/2
  Sum3/1 -> Sum2/2

== system fengji/Subsystem7/Subsystem6 ==
  In1 : Inport
  In2 : Inport  Port=2
  Bus Selector : BusSelector  OutputSignals=Stator current is_a (A),Stator current is_b (A),Stator current is_c (A)
  Bus Selector1 : BusSelector  OutputSignals=Rotor speed wm (rad/s),Rotor angle thetam (rad),Electromagnetic torque Te (N*m)
  Mux : Mux  Inputs=3
  iabc : Outport
  theta : Outport  Port=2
  Wm : Outport  Port=3
  Te : Outport  Port=4
  wires:
  In2/1 -> Bus Selector1/1
  In1/1 -> Bus Selector/1
  Bus Selector/3 -> Mux/3  "<Stator current is_c (A)>"
  Bus Selector/1 -> Mux/1  "<Stator current is_a (A)>"
  Bus Selector/2 -> Mux/2  "<Stator current is_b (A)>"
  Mux/1 -> iabc/1
  Bus Selector1/1 -> Wm/1  "<Rotor speed wm (rad/s)>"
  Bus Selector1/2 -> theta/1  "<Rotor angle thetam (rad)>"
  Bus Selector1/3 -> Te/1  "<Electromagnetic torque Te (N*m)>"

== system fengji/Subsystem7/anti_park ==
  Vq : Inport
  Vd : Inport  Port=2
  MATLAB Function : MATLAB Function  TreatAsAtomicUnit=on
  MATLAB Function1 : MATLAB Function  TreatAsAtomicUnit=on
  Mux : Mux  Inputs=3
  Ualpha : Outport
  Ubeta : Outport  Port=2
  wires:
  [the] -> Mux/1
  Vd/1 -> Mux/2
  Vq/1 -> Mux/3
  Mux/1 -> MATLAB Function1/1(u), MATLAB Function/1(u)
  MATLAB Function1/1(y) -> Ubeta/1
  MATLAB Function/1(y) -> Ualpha/1

== system fengji/Subsystem7/clark ==
  A : Inport
  B : Inport  Port=2
  C : Inport  Port=3
  MATLAB Function : MATLAB Function  TreatAsAtomicUnit=on
  MATLAB Function1 : MATLAB Function  TreatAsAtomicUnit=on
  Mux : Mux  Inputs=3
  Alpha : Outport
  Beta : Outport  Port=2
  wires:
  Mux/1 -> MATLAB Function1/1(u), MATLAB Function/1(u)
  MATLAB Function/1(y) -> Alpha/1
  B/1 -> Mux/2
  A/1 -> Mux/1
  C/1 -> Mux/3
  MATLAB Function1/1(y) -> Beta/1

== system fengji/Subsystem7/park ==
  Alpha1 : Inport
  Beta1 : Inport  Port=2
  theta : Inport  Port=3
  MATLAB Function : MATLAB Function  TreatAsAtomicUnit=on
  MATLAB Function1 : MATLAB Function  TreatAsAtomicUnit=on
  Mux : Mux  Inputs=3
  d : Outport
  q : Outport  Port=2
  wires:
  MATLAB Function1/1(y) -> q/1
  theta/1 -> Mux/3
  Alpha1/1 -> Mux/1
  Beta1/1 -> Mux/2
  MATLAB Function/1(y) -> d/1
  Mux/1 -> MATLAB Function/1(u), MATLAB Function1/1(u)

== system fengji/Subsystem7/svpwm' ==
  Uα : Inport
  Uβ : Inport  Port=2
  Scope2 : Scope  NumInputPorts=3
  Subsystem : Subsystem
  Subsystem1 : Subsystem
  Subsystem2 : Subsystem
  Subsystem3 : Subsystem
  Subsystem4 : Subsystem
  Subsystem5 : Subsystem
  Tpwm : Constant  Value=10e-5
  Udc : Constant  Value=Udc
  pwm : Subsystem
  svpwm : Outport
  wires:
  Subsystem4/2(Tb) -> Subsystem5/3(Tb), Scope2/2
  Subsystem1/1(N) -> Subsystem2/1(N), Subsystem5/1(N)
  Subsystem/2(Y) -> Subsystem2/3(Y)
  Subsystem2/1(T1) -> Subsystem3/1(T1)
  Subsystem3/1(T1') -> Subsystem4/1(T1')
  Subsystem3/2(T2') -> Subsystem4/2(T2')
  Uα/1 -> Subsystem1/1(Ualpha), Subsystem/1(Uα)
  Subsystem/1(X) -> Subsystem2/2(X)
  Subsystem/3(Z) -> Subsystem2/4(Z)
  Subsystem4/3(Tc) -> Scope2/3, Subsystem5/4(Tc)
  Uβ/1 -> Subsystem1/2(Ubeta), Subsystem/2(Uβ)
  Subsystem4/1(Ta) -> Scope2/1, Subsystem5/2(Ta)
  Subsystem2/2(T2) -> Subsystem3/2(T2)
  Udc/1 -> Subsystem/4(Udc)
  Tpwm/1 -> Subsystem4/3(Tpwm), Subsystem3/3(Tpwm), Subsystem/3(Tpwm)
  Subsystem5/1(Tcmp1) -> pwm/1(In1)
  Subsystem5/2(Tcmp2) -> pwm/2(In2)
  Subsystem5/3(Tcmp3) -> pwm/3(In3)
  pwm/1(Out1) -> svpwm/1

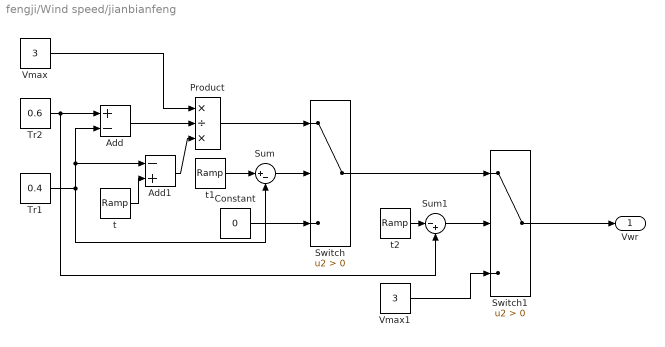
== system fengji/Wind speed/jianbianfeng ==
  Add : Sum  Inputs=+-
  Add1 : Sum  Inputs=-+
  Constant : Constant  Value=0
  Product : Product  Inputs=*/*
  Sum : Sum  Inputs=|+-
  Sum1 : Sum  Inputs=|-+
  Switch : Switch  Criteria=u2 > Threshold  SaturateOnIntegerOverflow=off  InputSameDT=off
  Switch1 : Switch  Criteria=u2 > Threshold  SaturateOnIntegerOverflow=off  InputSameDT=off
  Tr1 : Constant  Value=0.4
  Tr2 : Constant  Value=0.6
  Vmax : Constant  Value=3
  Vmax1 : Constant  Value=3
  t : simulink/Sources/Ramp  slope=1  start=0  InitialOutput=0
  t1 : simulink/Sources/Ramp  slope=1  start=0  InitialOutput=0
  t2 : simulink/Sources/Ramp  slope=1  start=0  InitialOutput=0
  Vwr : Outport
  wires:
  Tr1/1 -> Sum/2, Add1/1, Add/2
  Switch1/1 -> Vwr/1
  Switch/1 -> Switch1/1
  Sum1/1 -> Switch1/2
  Tr2/1 -> Sum1/2, Add/1
  t/1 -> Add1/2
  Product/1 -> Switch/1
  t2/1 -> Sum1/1
  t1/1 -> Sum/1
  Vmax/1 -> Product/1
  Vmax1/1 -> Switch1/3
  Constant/1 -> Switch/3
  Add1/1 -> Product/3
  Add/1 -> Product/2
  Sum/1 -> Switch/2

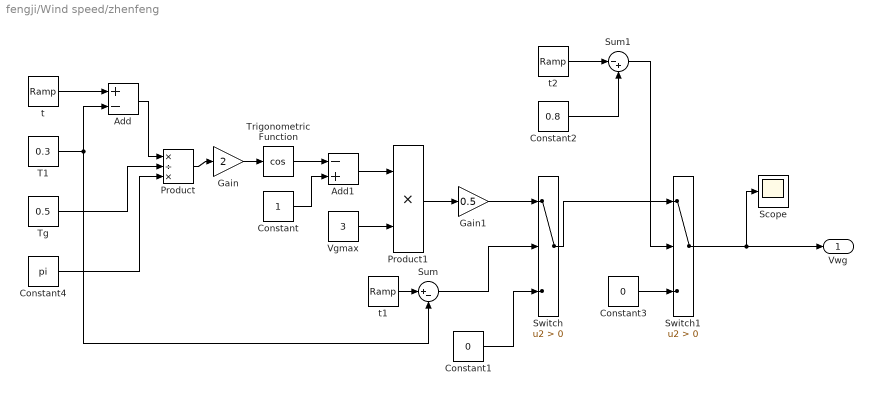
== system fengji/Wind speed/zhenfeng ==
  Add : Sum  Inputs=+-
  Add1 : Sum  Inputs=-+
  Constant : Constant
  Constant1 : Constant  Value=0
  Constant2 : Constant  Value=0.8
  Constant3 : Constant  Value=0
  Constant4 : Constant  Value=pi
  Gain : Gain  Gain=2
  Gain1 : Gain  Gain=0.5
  Product : Product  Inputs=*/*
  Product1 : Product
  Scope : Scope
  Sum : Sum  Inputs=|+-
  Sum1 : Sum  Inputs=|-+
  Switch : Switch  Criteria=u2 > Threshold  SaturateOnIntegerOverflow=off  InputSameDT=off
  Switch1 : Switch  Criteria=u2 > Threshold  SaturateOnIntegerOverflow=off  InputSameDT=off
  T1 : Constant  Value=0.3
  Tg : Constant  Value=0.5
  Trigonometric Function : Trigonometry  Operator=cos
  Vgmax : Constant  Value=3
  t : simulink/Sources/Ramp  slope=1  start=0  InitialOutput=0
  t1 : simulink/Sources/Ramp  slope=1  start=0  InitialOutput=0
  t2 : simulink/Sources/Ramp  slope=1  start=0  InitialOutput=0
  Vwg : Outport
  wires:
  Switch1/1 -> Vwg/1, Scope/1
  t1/1 -> Sum/1
  Constant/1 -> Add1/2
  T1/1 -> Sum/2, Add/2
  Sum1/1 -> Switch1/2
  Constant2/1 -> Sum1/2
  Add1/1 -> Product1/1
  Gain1/1 -> Switch/1
  Product1/1 -> Gain1/1
  Constant1/1 -> Switch/3
  Gain/1 -> Trigonometric Function/1
  Switch/1 -> Switch1/1
  Constant3/1 -> Switch1/3
  Sum/1 -> Switch/2
  t2/1 -> Sum1/1
  Product/1 -> Gain/1
  Add/1 -> Product/1
  Vgmax/1 -> Product1/2
  Trigonometric Function/1 -> Add1/1
  t/1 -> Add/1
  Tg/1 -> Product/2
  Constant4/1 -> Product/3

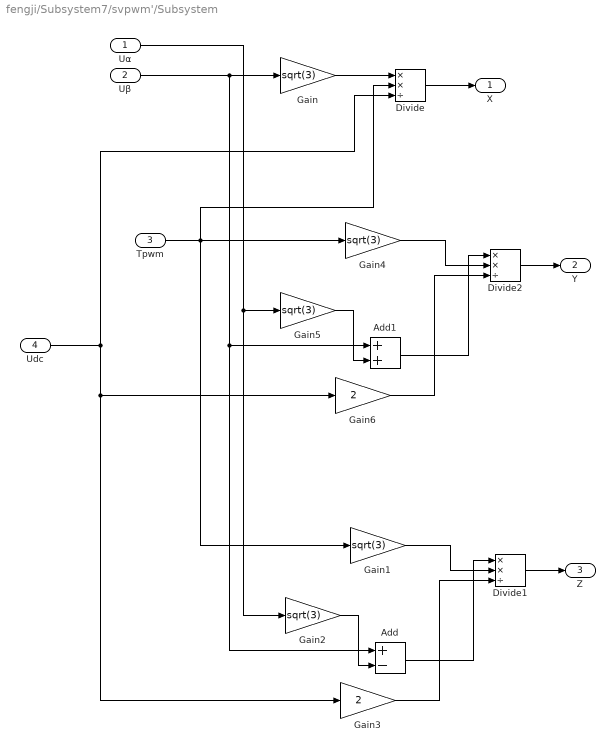
== system fengji/Subsystem7/svpwm'/Subsystem ==
  Uα : Inport
  Uβ : Inport  Port=2
  Tpwm : Inport  Port=3
  Udc : Inport  Port=4
  Add : Sum  Inputs=+-
  Add1 : Sum
  Divide : Product  Inputs=**/
  Divide1 : Product  Inputs=**/
  Divide2 : Product  Inputs=**/
  Gain{,1..2,4..5} (5 alike) : Gain  Gain=sqrt(3)
  Gain3 : Gain  Gain=2
  Gain6 : Gain  Gain=2
  X : Outport
  Y : Outport  Port=2
  Z : Outport  Port=3
  wires:
  Add/1 -> Divide1/1
  Tpwm/1 -> Gain1/1, Divide/2, Gain4/1
  Udc/1 -> Divide/3, Gain3/1, Gain6/1
  Uβ/1 -> Gain/1, Add1/1, Add/1
  Gain1/1 -> Divide1/2
  Gain2/1 -> Add/2
  Gain3/1 -> Divide1/3
  Divide/1 -> X/1
  Divide2/1 -> Y/1
  Uα/1 -> Gain5/1, Gain2/1
  Gain6/1 -> Divide2/3
  Gain4/1 -> Divide2/2
  Gain5/1 -> Add1/2
  Add1/1 -> Divide2/1
  Divide1/1 -> Z/1
  Gain/1 -> Divide/1

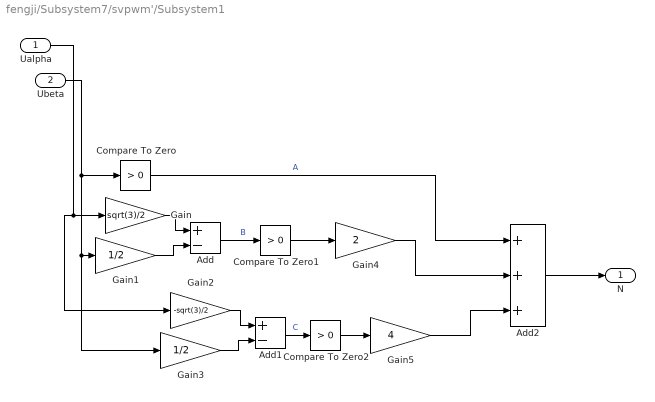
== system fengji/Subsystem7/svpwm'/Subsystem1 ==
  Ualpha : Inport
  Ubeta : Inport  Port=2
  Add : Sum  Inputs=+-
  Add1 : Sum  Inputs=+-
  Add2 : Sum  Inputs=+++
  Compare To Zero : simulink/Logic and Bit Operations/Compare To Zero  relop=>  OutDataTypeStr=boolean
  Compare To Zero1 : simulink/Logic and Bit Operations/Compare To Zero  relop=>  OutDataTypeStr=boolean
  Compare To Zero2 : simulink/Logic and Bit Operations/Compare To Zero  relop=>  OutDataTypeStr=boolean
  Gain : Gain  Gain=sqrt(3)/2
  Gain1 : Gain  Gain=1/2
  Gain2 : Gain  Gain=-sqrt(3)/2
  Gain3 : Gain  Gain=1/2
  Gain4 : Gain  Gain=2
  Gain5 : Gain  Gain=4
  N : Outport
  wires:
  Gain3/1 -> Add1/2
  Gain2/1 -> Add1/1
  Gain1/1 -> Add/2
  Add2/1 -> N/1
  Ualpha/1 -> Gain2/1, Gain/1
  Ubeta/1 -> Compare To Zero/1, Gain3/1, Gain1/1
  Compare To Zero/1 -> Add2/1  "A"
  Gain5/1 -> Add2/3
  Gain/1 -> Add/1
  Gain4/1 -> Add2/2
  Add/1 -> Compare To Zero1/1  "B"
  Compare To Zero1/1 -> Gain4/1
  Add1/1 -> Compare To Zero2/1  "C"
  Compare To Zero2/1 -> Gain5/1

== system fengji/Subsystem7/svpwm'/Subsystem2 ==
  N : Inport
  X : Inport  Port=2
  Y : Inport  Port=3
  Z : Inport  Port=4
  Gain{,1..3} (4 alike) : Gain  Gain=-1
  Multiport Switch : MultiPortSwitch  Inputs=6  SaturateOnIntegerOverflow=off  InputSameDT=off
  Multiport Switch1 : MultiPortSwitch  Inputs=6  SaturateOnIntegerOverflow=off  InputSameDT=off
  T1 : Outport
  T2 : Outport  Port=2
  wires:
  Gain2/1 -> Multiport Switch1/7, Multiport Switch/6
  Z/1 -> Gain3/1, Multiport Switch/5, Multiport Switch1/2, Gain1/1
  Gain1/1 -> Multiport Switch1/4
  Multiport Switch1/1 -> T1/1
  N/1 -> Multiport Switch1/1, Multiport Switch/1
  X/1 -> Multiport Switch1/6, Multiport Switch/4, Gain/1
  Multiport Switch/1 -> T2/1
  Gain3/1 -> Multiport Switch/7
  Y/1 -> Gain2/1, Multiport Switch1/3, Multiport Switch/2
  Gain/1 -> Multiport Switch1/5, Multiport Switch/3

== system fengji/Subsystem7/svpwm'/Subsystem3 ==
  T1 : Inport
  T2 : Inport  Port=2
  Tpwm : Inport  Port=3
  Add : Sum
  Divide : Product  Inputs=**/
  Divide1 : Product  Inputs=**/
  Relational Operator : RelationalOperator  Operator=>  OutDataTypeStr=boolean  InputSameDT=off
  Switch : Switch  Criteria=u2 > Threshold  SaturateOnIntegerOverflow=off  InputSameDT=off
  Switch1 : Switch  Criteria=u2 > Threshold  SaturateOnIntegerOverflow=off  InputSameDT=off
  T1' : Outport
  T2' : Outport  Port=2
  wires:
  Tpwm/1 -> Divide1/2, Divide/2, Relational Operator/2
  Divide1/1 -> Switch1/1
  T1/1 -> Divide/1, Switch/3, Add/1
  Switch1/1 -> T2'/1
  T2/1 -> Divide1/1, Switch1/3, Add/2
  Switch/1 -> T1'/1
  Divide/1 -> Switch/1
  Add/1 -> Divide1/3, Divide/3, Relational Operator/1
  Relational Operator/1 -> Switch1/2, Switch/2
